simulink model "ThdRwLtStBkReclnIsPosChk"  (R2024b)
settings: Solver=FixedStepDiscrete  StartTime=0.0  StopTime=10.0  FixedStep=0.01  RelTol=1e-3
undefined symbols (not defined in the file or in its folder): KeSMSuThrdRwStBackPosDelta_Val, KeSMSuThrdRwStBackPosTolr_Val, KeSMSuVehicleModelConfig_Val
libraries: StIsPosChkLib x14, simulink x5
(part 1 of 2)
settings Model: Creator=sn2xws  LastModifiedBy=sn55gm
settings Model: ModifiedHistory=|
  | 2024.3.14
  | V2.3.0
  | Bug 813950 童锁Lock，Mode1_Easy Entry Mode 不应调用失败
  | 2024.6.25
  | V3.0.0 557模式流程V1.6
  | 
  | 2024.7.5
  | V3.0.0 557模式流程V1.9
  | 2024.9.5 V3.0.1 新增Md56
  | 2024.10.14 V3.0.2 新增Md57 Md58
  | 2024.10.28 V3.0.3 6s不选Md12目标位置
  | 2024.11.11 V3.0.4 vip模式到位置不看三排
  | 2024.12.24 V3.8.0 CR960542 7s智享退出模式左右同时调用时，三排座椅前后记忆位置使用逻辑
  | 2025.2.19 V3.8.1 Bug 991386 Md1 三排占座时未移动且报了成功
  | 25.6.30 V3.13.0 新增Md61 md62
settings SolverCC: AlgebraicLoopSolver=TrustRegion
settings DataIOCC: SaveFormat=StructureWithTime  ReturnWorkspaceOutputs=off
settings OptimizationCC: DefaultParameterBehavior=Inlined  EnhancedBackFolding=on  PassReuseOutputArgsAs=Individual arguments  ZeroExternalMemoryAtStartup=off  ZeroInternalMemoryAtStartup=off  OptimizeBlockOrder=speed  DifferentSizesBufferReuse=on  OptimizationCustomize=off  EfficientTunableParamExpr=on
settings DebuggingCC: ParameterTunabilityLossMsg=error  UnconnectedInputMsg=warning  UnconnectedOutputMsg=warning  UnconnectedLineMsg=warning  ArithmeticOperatorsInVariantConditions=warning
settings ModelReferenceCC: EnableRefExpFcnMdlSchedulingChecks=on  ModelReferenceNumInstancesAllowed=Single
settings SFSimCC: MATLABDynamicMemAlloc=off  CustomCodeUndefinedFunction=UseInterfaceOnly
settings RTWCC: Description=AUTOSAR  SystemTargetFile=autosar.tlc  GenCodeOnly=on  TemplateMakefile=ert_default_tmf  GenerateReport=on  IncludeHyperlinkInReport=on  LaunchReport=on  DataTypeReplacement=CDataTypesFixedWidth  GenerateTraceInfo=on  GenerateTraceReport=on  GenerateTraceReportSl=on  GenerateTraceReportSf=on  GenerateTraceReportEml=on  GPUComputeCapability=3.5
settings CodeAppCC: ForceParamTrailComments=on  IgnoreCustomStorageClasses=off  OperatorAnnotations=on  SimulinkDataObjDesc=on  SFDataObjDesc=on  InsertBlockDesc=on
settings STFCustomTargetCC: TargetLangStandard=C99 (ISO)  MultiwordLength=256  ParMdlRefBuildCompliant=on  CompOptLevelCompliant=on  IncludeMdlTerminateFcn=off  CombineOutputUpdateFcns=on  SuppressErrorStatus=on  ERTCustomFileBanners=on  SupportNonFinite=off  SupportComplex=off  SupportContinuousTime=off  SupportNonInlinedSFcns=off  RemoveResetFunc=on  MATLABClassNameForMDSCustomization=Simulink.SoftwareTarget.ERTCustomization  AutosarCompliant=on  UseToolchainInfoCompliant=on  LookupTableObjectStructAxisOrder=2,1,3,4,...  LUTObjectStructOrderEvenSpacing=Size,Table,Breakpoints  SystemTargetFile=autosar.tlc
settings ERTTargetCC: TargetLangStandard=C99 (ISO)  ConcurrentExecutionCompliant=off  IncludeMdlTerminateFcn=off  SuppressErrorStatus=on  SupportNonFinite=off  SupportComplex=off  ModelStepFunctionPrototypeControlCompliant=off  CPPClassGenCompliant=off  AutosarCompliant=on  LookupTableObjectStructAxisOrder=2,1,3,4,...  LUTObjectStructOrderEvenSpacing=Size,Table,Breakpoints  ERTCustomFileTemplate=example_file_process.tlc  ERTFilePackagingFormat=Compact  BooleanTrueId=TRUE  BooleanFalseId=FALSE  DynamicArrayContainerType=coder::array

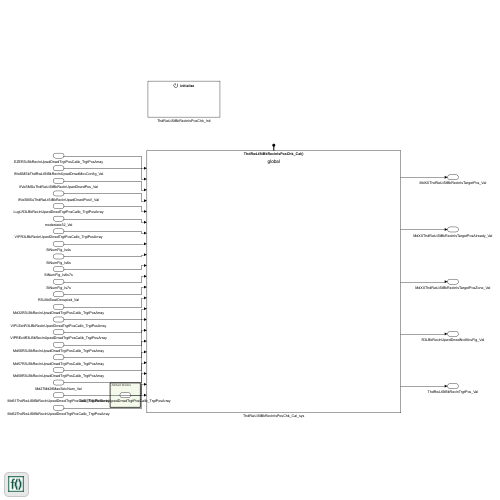
[thumbnail: Simulink's stored preview of the top-level diagram]
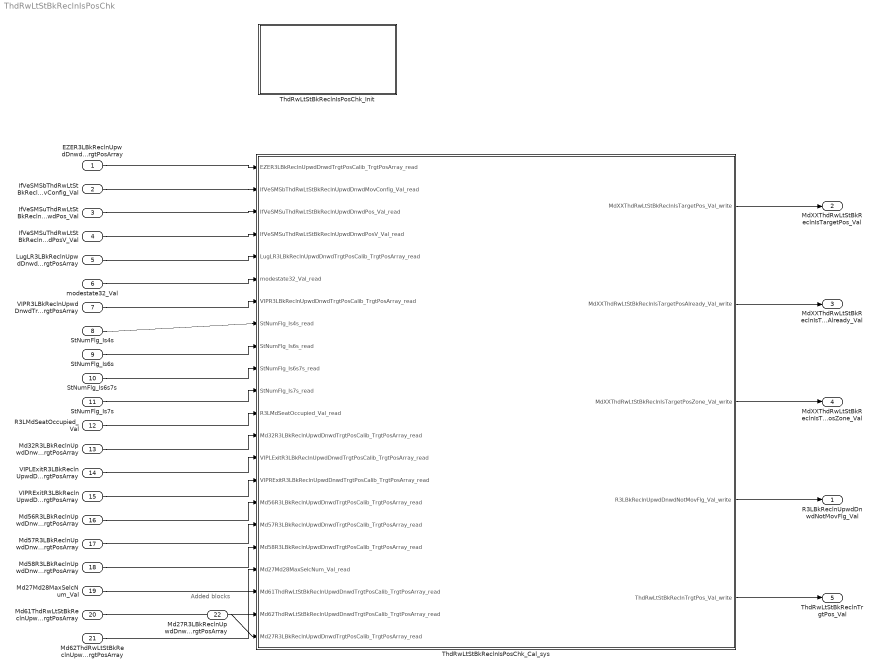
== system ThdRwLtStBkReclnIsPosChk ==
  note: Added blocks
  EZER3LBkReclnUpwdDnwdTrgtPosCalib_TrgtPosArray : Inport  Description=|  OutDataTypeStr=uint16  PortDimensions=3
      | 0:Pos
      | 1:Max
      | 2:Min
  IfVeSMSbThdRwLtStBkReclnUpwdDnwdMovConfig_Val : Inport  Port=2  OutDataTypeStr=boolean  PortDimensions=1
  IfVeSMSuThdRwLtStBkReclnUpwdDnwdPos_Val : Inport  Port=3  OutDataTypeStr=uint16  PortDimensions=1
  IfVeSMSuThdRwLtStBkReclnUpwdDnwdPosV_Val : Inport  Port=4  OutDataTypeStr=boolean  PortDimensions=1
  LugLR3LBkReclnUpwdDnwdTrgtPosCalib_TrgtPosArray : Inport  Description=|  Port=5  OutDataTypeStr=uint16  PortDimensions=3
      | 0:Pos
      | 1:Max
      | 2:Min
  modestate32_Val : Inport  Port=6  OutDataTypeStr=uint32  PortDimensions=1
  VIPR3LBkReclnUpwdDnwdTrgtPosCalib_TrgtPosArray : Inport  Description=|  Port=7  OutDataTypeStr=uint16  PortDimensions=3
      | 0:Pos
      | 1:Max
      | 2:Min
  StNumFlg_Is4s : Inport  Port=8  OutDataTypeStr=boolean  PortDimensions=1
  StNumFlg_Is6s : Inport  Port=9  OutDataTypeStr=boolean  PortDimensions=1
  StNumFlg_Is6s7s : Inport  Port=10  OutDataTypeStr=boolean  PortDimensions=1
  StNumFlg_Is7s : Inport  Port=11  OutDataTypeStr=boolean  PortDimensions=1
  R3LMdSeatOccupied_Val : Inport  Port=12  OutDataTypeStr=boolean  PortDimensions=1
  Md32R3LBkReclnUpwdDnwdTrgtPosCalib_TrgtPosArray : Inport  Description=|  Port=13  OutDataTypeStr=uint16  PortDimensions=3
      | 0:Pos
      | 1:Max
      | 2:Min
  VIPLExitR3LBkReclnUpwdDnwdTrgtPosCalib_TrgtPosArray : Inport  Description=|  Port=14  OutDataTypeStr=uint16  PortDimensions=3
      | 0:Pos
      | 1:Max
      | 2:Min
  VIPRExitR3LBkReclnUpwdDnwdTrgtPosCalib_TrgtPosArray : Inport  Description=|  Port=15  OutDataTypeStr=uint16  PortDimensions=3
      | 0:Pos
      | 1:Max
      | 2:Min
  Md56R3LBkReclnUpwdDnwdTrgtPosCalib_TrgtPosArray : Inport  Description=|  Port=16  OutDataTypeStr=uint16  PortDimensions=3
      | 0:Pos
      | 1:Max
      | 2:Min
  Md57R3LBkReclnUpwdDnwdTrgtPosCalib_TrgtPosArray : Inport  Description=|  Port=17  OutDataTypeStr=uint16  PortDimensions=3
      | 0:Pos
      | 1:Max
      | 2:Min
  Md58R3LBkReclnUpwdDnwdTrgtPosCalib_TrgtPosArray : Inport  Description=|  Port=18  OutDataTypeStr=uint16  PortDimensions=3
      | 0:Pos
      | 1:Max
      | 2:Min
  Md27Md28MaxSelcNum_Val : Inport  Port=19  OutDataTypeStr=uint8  PortDimensions=1
  Md61ThdRwLtStBkReclnUpwdDnwdTrgtPosCalib_TrgtPosArray : Inport  Description=|  Port=20  OutDataTypeStr=uint16  PortDimensions=3
      | 0:Pos
      | 1:Max
      | 2:Min
  Md62ThdRwLtStBkReclnUpwdDnwdTrgtPosCalib_TrgtPosArray : Inport  Description=|  Port=21  OutDataTypeStr=uint16  PortDimensions=3
      | 0:Pos
      | 1:Max
      | 2:Min
  Md27R3LBkReclnUpwdDnwdTrgtPosCalib_TrgtPosArray : Inport  Description=|  Port=22  OutDataTypeStr=uint16  PortDimensions=3
      | 0:Pos
      | 1:Max
      | 2:Min
  ThdRwLtStBkReclnIsPosChk_Cal_sys : Subsystem
  ThdRwLtStBkReclnIsPosChk_Init : Subsystem
  R3LBkReclnUpwdDnwdNotMovFlg_Val : Outport  OutDataTypeStr=boolean  PortDimensions=1  VectorParamsAs1DForOutWhenUnconnected=off
  MdXXThdRwLtStBkReclnIsTargetPos_Val : Outport  Port=2  OutDataTypeStr=uint32  PortDimensions=1  VectorParamsAs1DForOutWhenUnconnected=off
  MdXXThdRwLtStBkReclnIsTargetPosAlready_Val : Outport  Port=3  OutDataTypeStr=uint32  PortDimensions=1  VectorParamsAs1DForOutWhenUnconnected=off
  MdXXThdRwLtStBkReclnIsTargetPosZone_Val : Outport  Port=4  OutDataTypeStr=uint32  PortDimensions=1  VectorParamsAs1DForOutWhenUnconnected=off
  ThdRwLtStBkReclnTrgtPos_Val : Outport  Port=5  OutDataTypeStr=uint16  PortDimensions=1  VectorParamsAs1DForOutWhenUnconnected=off
  wires:
  EZER3LBkReclnUpwdDnwdTrgtPosCalib_TrgtPosArray/1 -> ThdRwLtStBkReclnIsPosChk_Cal_sys/1(EZER3LBkReclnUpwdDnwdTrgtPosCalib_TrgtPosArray_read)
  IfVeSMSbThdRwLtStBkReclnUpwdDnwdMovConfig_Val/1 -> ThdRwLtStBkReclnIsPosChk_Cal_sys/2(IfVeSMSbThdRwLtStBkReclnUpwdDnwdMovConfig_Val_read)
  IfVeSMSuThdRwLtStBkReclnUpwdDnwdPos_Val/1 -> ThdRwLtStBkReclnIsPosChk_Cal_sys/3(IfVeSMSuThdRwLtStBkReclnUpwdDnwdPos_Val_read)
  IfVeSMSuThdRwLtStBkReclnUpwdDnwdPosV_Val/1 -> ThdRwLtStBkReclnIsPosChk_Cal_sys/4(IfVeSMSuThdRwLtStBkReclnUpwdDnwdPosV_Val_read)
  LugLR3LBkReclnUpwdDnwdTrgtPosCalib_TrgtPosArray/1 -> ThdRwLtStBkReclnIsPosChk_Cal_sys/5(LugLR3LBkReclnUpwdDnwdTrgtPosCalib_TrgtPosArray_read)
  modestate32_Val/1 -> ThdRwLtStBkReclnIsPosChk_Cal_sys/6(modestate32_Val_read)
  VIPR3LBkReclnUpwdDnwdTrgtPosCalib_TrgtPosArray/1 -> ThdRwLtStBkReclnIsPosChk_Cal_sys/7(VIPR3LBkReclnUpwdDnwdTrgtPosCalib_TrgtPosArray_read)
  ThdRwLtStBkReclnIsPosChk_Cal_sys/1(MdXXThdRwLtStBkReclnIsTargetPos_Val_write) -> MdXXThdRwLtStBkReclnIsTargetPos_Val/1
  ThdRwLtStBkReclnIsPosChk_Cal_sys/2(MdXXThdRwLtStBkReclnIsTargetPosAlready_Val_write) -> MdXXThdRwLtStBkReclnIsTargetPosAlready_Val/1
  ThdRwLtStBkReclnIsPosChk_Cal_sys/3(MdXXThdRwLtStBkReclnIsTargetPosZone_Val_write) -> MdXXThdRwLtStBkReclnIsTargetPosZone_Val/1
  ThdRwLtStBkReclnIsPosChk_Cal_sys/4(R3LBkReclnUpwdDnwdNotMovFlg_Val_write) -> R3LBkReclnUpwdDnwdNotMovFlg_Val/1
  ThdRwLtStBkReclnIsPosChk_Cal_sys/5(ThdRwLtStBkReclnTrgtPos_Val_write) -> ThdRwLtStBkReclnTrgtPos_Val/1
  StNumFlg_Is4s/1 -> ThdRwLtStBkReclnIsPosChk_Cal_sys/8(StNumFlg_Is4s_read)
  StNumFlg_Is6s/1 -> ThdRwLtStBkReclnIsPosChk_Cal_sys/9(StNumFlg_Is6s_read)
  StNumFlg_Is6s7s/1 -> ThdRwLtStBkReclnIsPosChk_Cal_sys/10(StNumFlg_Is6s7s_read)
  StNumFlg_Is7s/1 -> ThdRwLtStBkReclnIsPosChk_Cal_sys/11(StNumFlg_Is7s_read)
  R3LMdSeatOccupied_Val/1 -> ThdRwLtStBkReclnIsPosChk_Cal_sys/12(R3LMdSeatOccupied_Val_read)
  Md32R3LBkReclnUpwdDnwdTrgtPosCalib_TrgtPosArray/1 -> ThdRwLtStBkReclnIsPosChk_Cal_sys/13(Md32R3LBkReclnUpwdDnwdTrgtPosCalib_TrgtPosArray_read)
  VIPLExitR3LBkReclnUpwdDnwdTrgtPosCalib_TrgtPosArray/1 -> ThdRwLtStBkReclnIsPosChk_Cal_sys/14(VIPLExitR3LBkReclnUpwdDnwdTrgtPosCalib_TrgtPosArray_read)
  VIPRExitR3LBkReclnUpwdDnwdTrgtPosCalib_TrgtPosArray/1 -> ThdRwLtStBkReclnIsPosChk_Cal_sys/15(VIPRExitR3LBkReclnUpwdDnwdTrgtPosCalib_TrgtPosArray_read)
  Md56R3LBkReclnUpwdDnwdTrgtPosCalib_TrgtPosArray/1 -> ThdRwLtStBkReclnIsPosChk_Cal_sys/16(Md56R3LBkReclnUpwdDnwdTrgtPosCalib_TrgtPosArray_read)
  Md57R3LBkReclnUpwdDnwdTrgtPosCalib_TrgtPosArray/1 -> ThdRwLtStBkReclnIsPosChk_Cal_sys/17(Md57R3LBkReclnUpwdDnwdTrgtPosCalib_TrgtPosArray_read)
  Md58R3LBkReclnUpwdDnwdTrgtPosCalib_TrgtPosArray/1 -> ThdRwLtStBkReclnIsPosChk_Cal_sys/18(Md58R3LBkReclnUpwdDnwdTrgtPosCalib_TrgtPosArray_read)
  Md27Md28MaxSelcNum_Val/1 -> ThdRwLtStBkReclnIsPosChk_Cal_sys/19(Md27Md28MaxSelcNum_Val_read)
  Md61ThdRwLtStBkReclnUpwdDnwdTrgtPosCalib_TrgtPosArray/1 -> ThdRwLtStBkReclnIsPosChk_Cal_sys/20(Md61ThdRwLtStBkReclnUpwdDnwdTrgtPosCalib_TrgtPosArray_read)
  Md62ThdRwLtStBkReclnUpwdDnwdTrgtPosCalib_TrgtPosArray/1 -> ThdRwLtStBkReclnIsPosChk_Cal_sys/21(Md62ThdRwLtStBkReclnUpwdDnwdTrgtPosCalib_TrgtPosArray_read)
  Md27R3LBkReclnUpwdDnwdTrgtPosCalib_TrgtPosArray/1 -> ThdRwLtStBkReclnIsPosChk_Cal_sys/22(Md27R3LBkReclnUpwdDnwdTrgtPosCalib_TrgtPosArray_read)

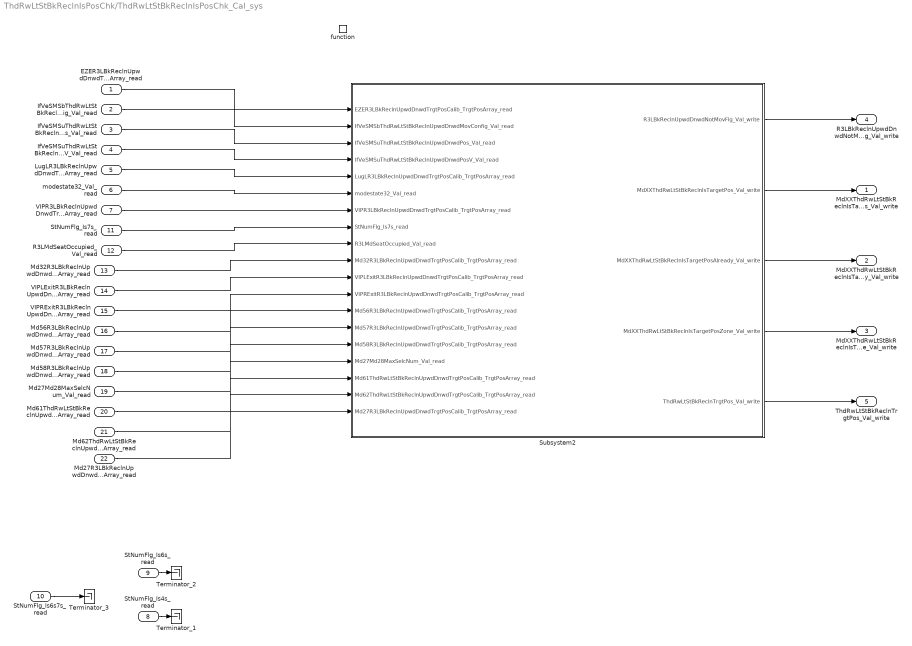
== system ThdRwLtStBkReclnIsPosChk/ThdRwLtStBkReclnIsPosChk_Cal_sys ==
  EZER3LBkReclnUpwdDnwdTrgtPosCalib_TrgtPosArray_read : Inport
  IfVeSMSbThdRwLtStBkReclnUpwdDnwdMovConfig_Val_read : Inport  Port=2
  IfVeSMSuThdRwLtStBkReclnUpwdDnwdPos_Val_read : Inport  Port=3
  IfVeSMSuThdRwLtStBkReclnUpwdDnwdPosV_Val_read : Inport  Port=4
  LugLR3LBkReclnUpwdDnwdTrgtPosCalib_TrgtPosArray_read : Inport  Port=5
  modestate32_Val_read : Inport  Port=6
  VIPR3LBkReclnUpwdDnwdTrgtPosCalib_TrgtPosArray_read : Inport  Port=7
  StNumFlg_Is4s_read : Inport  Port=8
  StNumFlg_Is6s_read : Inport  Port=9
  StNumFlg_Is6s7s_read : Inport  Port=10
  StNumFlg_Is7s_read : Inport  Port=11
  R3LMdSeatOccupied_Val_read : Inport  Port=12
  Md32R3LBkReclnUpwdDnwdTrgtPosCalib_TrgtPosArray_read : Inport  Port=13
  VIPLExitR3LBkReclnUpwdDnwdTrgtPosCalib_TrgtPosArray_read : Inport  Port=14
  VIPRExitR3LBkReclnUpwdDnwdTrgtPosCalib_TrgtPosArray_read : Inport  Port=15
  Md56R3LBkReclnUpwdDnwdTrgtPosCalib_TrgtPosArray_read : Inport  Port=16
  Md57R3LBkReclnUpwdDnwdTrgtPosCalib_TrgtPosArray_read : Inport  Port=17
  Md58R3LBkReclnUpwdDnwdTrgtPosCalib_TrgtPosArray_read : Inport  Port=18
  Md27Md28MaxSelcNum_Val_read : Inport  Port=19
  Md61ThdRwLtStBkReclnUpwdDnwdTrgtPosCalib_TrgtPosArray_read : Inport  Port=20
  Md62ThdRwLtStBkReclnUpwdDnwdTrgtPosCalib_TrgtPosArray_read : Inport  Port=21
  Md27R3LBkReclnUpwdDnwdTrgtPosCalib_TrgtPosArray_read : Inport  Port=22
  function : TriggerPort  TriggerType=function-call  IsSimulinkFunction=on  FunctionName=ThdRwLtStBkReclnIsPosChk_Cal  VariantControl=(inherit)
  Subsystem2 : Subsystem
  Terminator_1 : Terminator
  Terminator_2 : Terminator
  Terminator_3 : Terminator
  MdXXThdRwLtStBkReclnIsTargetPos_Val_write : Outport  VectorParamsAs1DForOutWhenUnconnected=off
      settings: EnsureOutportIsVirtual=on
  MdXXThdRwLtStBkReclnIsTargetPosAlready_Val_write : Outport  Port=2  VectorParamsAs1DForOutWhenUnconnected=off
      settings: EnsureOutportIsVirtual=on
  MdXXThdRwLtStBkReclnIsTargetPosZone_Val_write : Outport  Port=3  VectorParamsAs1DForOutWhenUnconnected=off
      settings: EnsureOutportIsVirtual=on
  R3LBkReclnUpwdDnwdNotMovFlg_Val_write : Outport  Port=4  VectorParamsAs1DForOutWhenUnconnected=off
      settings: EnsureOutportIsVirtual=on
  ThdRwLtStBkReclnTrgtPos_Val_write : Outport  Port=5  VectorParamsAs1DForOutWhenUnconnected=off
      settings: EnsureOutportIsVirtual=on
  wires:
  Subsystem2/1(R3LBkReclnUpwdDnwdNotMovFlg_Val_write) -> R3LBkReclnUpwdDnwdNotMovFlg_Val_write/1
  Subsystem2/2(MdXXThdRwLtStBkReclnIsTargetPos_Val_write) -> MdXXThdRwLtStBkReclnIsTargetPos_Val_write/1
  Subsystem2/3(MdXXThdRwLtStBkReclnIsTargetPosAlready_Val_write) -> MdXXThdRwLtStBkReclnIsTargetPosAlready_Val_write/1
  Subsystem2/4(MdXXThdRwLtStBkReclnIsTargetPosZone_Val_write) -> MdXXThdRwLtStBkReclnIsTargetPosZone_Val_write/1
  Subsystem2/5(ThdRwLtStBkReclnTrgtPos_Val_write) -> ThdRwLtStBkReclnTrgtPos_Val_write/1
  IfVeSMSuThdRwLtStBkReclnUpwdDnwdPos_Val_read/1 -> Subsystem2/3(IfVeSMSuThdRwLtStBkReclnUpwdDnwdPos_Val_read)
  IfVeSMSbThdRwLtStBkReclnUpwdDnwdMovConfig_Val_read/1 -> Subsystem2/2(IfVeSMSbThdRwLtStBkReclnUpwdDnwdMovConfig_Val_read)
  EZER3LBkReclnUpwdDnwdTrgtPosCalib_TrgtPosArray_read/1 -> Subsystem2/1(EZER3LBkReclnUpwdDnwdTrgtPosCalib_TrgtPosArray_read)
  IfVeSMSuThdRwLtStBkReclnUpwdDnwdPosV_Val_read/1 -> Subsystem2/4(IfVeSMSuThdRwLtStBkReclnUpwdDnwdPosV_Val_read)
  LugLR3LBkReclnUpwdDnwdTrgtPosCalib_TrgtPosArray_read/1 -> Subsystem2/5(LugLR3LBkReclnUpwdDnwdTrgtPosCalib_TrgtPosArray_read)
  modestate32_Val_read/1 -> Subsystem2/6(modestate32_Val_read)
  VIPR3LBkReclnUpwdDnwdTrgtPosCalib_TrgtPosArray_read/1 -> Subsystem2/7(VIPR3LBkReclnUpwdDnwdTrgtPosCalib_TrgtPosArray_read)
  StNumFlg_Is4s_read/1 -> Terminator_1/1
  StNumFlg_Is6s7s_read/1 -> Terminator_3/1
  StNumFlg_Is7s_read/1 -> Subsystem2/8(StNumFlg_Is7s_read)
  StNumFlg_Is6s_read/1 -> Terminator_2/1
  R3LMdSeatOccupied_Val_read/1 -> Subsystem2/9(R3LMdSeatOccupied_Val_read)
  Md32R3LBkReclnUpwdDnwdTrgtPosCalib_TrgtPosArray_read/1 -> Subsystem2/10(Md32R3LBkReclnUpwdDnwdTrgtPosCalib_TrgtPosArray_read)
  VIPLExitR3LBkReclnUpwdDnwdTrgtPosCalib_TrgtPosArray_read/1 -> Subsystem2/11(VIPLExitR3LBkReclnUpwdDnwdTrgtPosCalib_TrgtPosArray_read)
  VIPRExitR3LBkReclnUpwdDnwdTrgtPosCalib_TrgtPosArray_read/1 -> Subsystem2/12(VIPRExitR3LBkReclnUpwdDnwdTrgtPosCalib_TrgtPosArray_read)
  Md56R3LBkReclnUpwdDnwdTrgtPosCalib_TrgtPosArray_read/1 -> Subsystem2/13(Md56R3LBkReclnUpwdDnwdTrgtPosCalib_TrgtPosArray_read)
  Md57R3LBkReclnUpwdDnwdTrgtPosCalib_TrgtPosArray_read/1 -> Subsystem2/14(Md57R3LBkReclnUpwdDnwdTrgtPosCalib_TrgtPosArray_read)
  Md58R3LBkReclnUpwdDnwdTrgtPosCalib_TrgtPosArray_read/1 -> Subsystem2/15(Md58R3LBkReclnUpwdDnwdTrgtPosCalib_TrgtPosArray_read)
  Md27Md28MaxSelcNum_Val_read/1 -> Subsystem2/16(Md27Md28MaxSelcNum_Val_read)
  Md61ThdRwLtStBkReclnUpwdDnwdTrgtPosCalib_TrgtPosArray_read/1 -> Subsystem2/17(Md61ThdRwLtStBkReclnUpwdDnwdTrgtPosCalib_TrgtPosArray_read)
  Md62ThdRwLtStBkReclnUpwdDnwdTrgtPosCalib_TrgtPosArray_read/1 -> Subsystem2/18(Md62ThdRwLtStBkReclnUpwdDnwdTrgtPosCalib_TrgtPosArray_read)
  Md27R3LBkReclnUpwdDnwdTrgtPosCalib_TrgtPosArray_read/1 -> Subsystem2/19(Md27R3LBkReclnUpwdDnwdTrgtPosCalib_TrgtPosArray_read)

== system ThdRwLtStBkReclnIsPosChk/ThdRwLtStBkReclnIsPosChk_Init ==
  note: Added blocks
  note: Added blocks
  note: Added blocks
  Event Listener : EventListener  EventName=reset
  PA_KeSMSuThrdRwStBackPosDelta_Val : Constant  Value=KeSMSuThrdRwStBackPosDelta_Val
  PA_KeSMSuThrdRwStBackPosTolr_Val : Constant  Value=KeSMSuThrdRwStBackPosTolr_Val
  PA_KeSMSuVehicleModelConfig_Val : Constant  Value=KeSMSuVehicleModelConfig_Val
  Terminator_1 : Terminator
  Terminator_2 : Terminator
  Terminator_3 : Terminator
  wires:
  PA_KeSMSuThrdRwStBackPosDelta_Val/1 -> Terminator_1/1
  PA_KeSMSuThrdRwStBackPosTolr_Val/1 -> Terminator_2/1
  PA_KeSMSuVehicleModelConfig_Val/1 -> Terminator_3/1

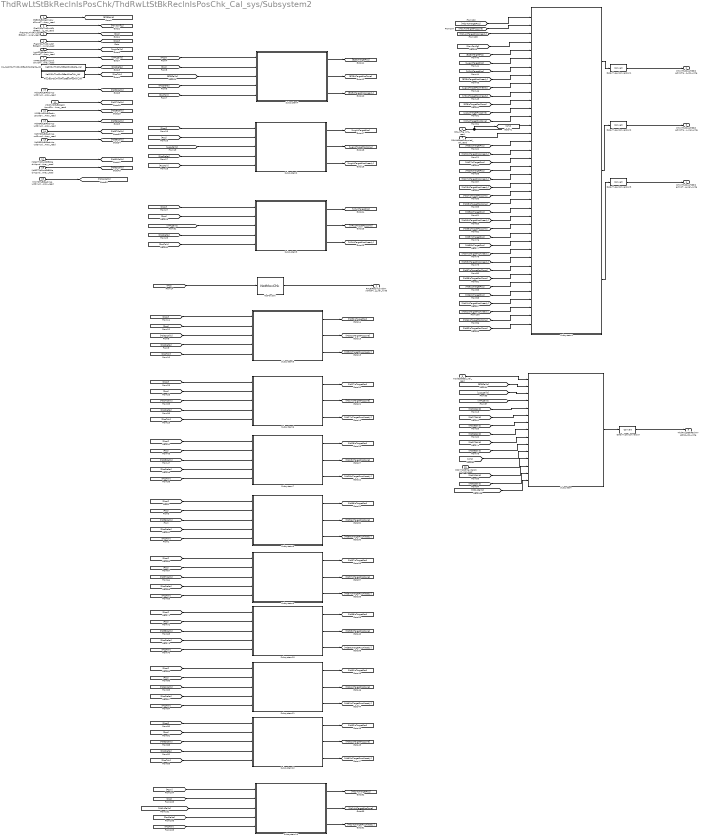
== system ThdRwLtStBkReclnIsPosChk/ThdRwLtStBkReclnIsPosChk_Cal_sys/Subsystem2 ==
  EZER3LBkReclnUpwdDnwdTrgtPosCalib_TrgtPosArray_read : Inport
  IfVeSMSbThdRwLtStBkReclnUpwdDnwdMovConfig_Val_read : Inport  Port=2
  IfVeSMSuThdRwLtStBkReclnUpwdDnwdPos_Val_read : Inport  Port=3
  IfVeSMSuThdRwLtStBkReclnUpwdDnwdPosV_Val_read : Inport  Port=4
  LugLR3LBkReclnUpwdDnwdTrgtPosCalib_TrgtPosArray_read : Inport  Port=5
  modestate32_Val_read : Inport  Port=6
  VIPR3LBkReclnUpwdDnwdTrgtPosCalib_TrgtPosArray_read : Inport  Port=7
  StNumFlg_Is7s_read : Inport  Port=8
  R3LMdSeatOccupied_Val_read : Inport  Port=9
  Md32R3LBkReclnUpwdDnwdTrgtPosCalib_TrgtPosArray_read : Inport  Port=10
  VIPLExitR3LBkReclnUpwdDnwdTrgtPosCalib_TrgtPosArray_read : Inport  Port=11
  VIPRExitR3LBkReclnUpwdDnwdTrgtPosCalib_TrgtPosArray_read : Inport  Port=12
  Md56R3LBkReclnUpwdDnwdTrgtPosCalib_TrgtPosArray_read : Inport  Port=13
  Md57R3LBkReclnUpwdDnwdTrgtPosCalib_TrgtPosArray_read : Inport  Port=14
  Md58R3LBkReclnUpwdDnwdTrgtPosCalib_TrgtPosArray_read : Inport  Port=15
  Md27Md28MaxSelcNum_Val_read : Inport  Port=16
  Md61ThdRwLtStBkReclnUpwdDnwdTrgtPosCalib_TrgtPosArray_read : Inport  Port=17
  Md62ThdRwLtStBkReclnUpwdDnwdTrgtPosCalib_TrgtPosArray_read : Inport  Port=18
  Md27R3LBkReclnUpwdDnwdTrgtPosCalib_TrgtPosArray_read : Inport  Port=19
  Data Type Conversion{,1..3} (4 alike) : DataTypeConversion  SaturateOnIntegerOverflow=off  RndMeth=Floor
  NotMovChk : StIsPosChkLib/NotMovChk  SystemSampleTime=-1  VariantActivationTime=update diagram  AllowFlexibleInterface=on  Latency=0  AutoFrameSizeCalculation=off
  PA_KeSMSuThrdRwStBackPosDelta_Val : Constant  Value=KeSMSuThrdRwStBackPosDelta_Val
  PA_KeSMSuThrdRwStBackPosTolr_Val : Constant  Value=KeSMSuThrdRwStBackPosTolr_Val
  Subsystem : Subsystem
  Subsystem1 : Subsystem
  Subsystem10 : Subsystem
  Subsystem11 : Subsystem
  Subsystem12 : Subsystem
  Subsystem13 : Subsystem
  Subsystem2 : Subsystem
  Subsystem3 : Subsystem
  Subsystem4 : Subsystem
  Subsystem5 : Subsystem
  Subsystem6 : Subsystem
  Subsystem7 : Subsystem
  Subsystem8 : Subsystem
  Subsystem9 : Subsystem
  R3LBkReclnUpwdDnwdNotMovFlg_Val_write : Outport  VectorParamsAs1DForOutWhenUnconnected=off
      settings: EnsureOutportIsVirtual=on
  MdXXThdRwLtStBkReclnIsTargetPos_Val_write : Outport  Port=2  VectorParamsAs1DForOutWhenUnconnected=off
      settings: EnsureOutportIsVirtual=on
  MdXXThdRwLtStBkReclnIsTargetPosAlready_Val_write : Outport  Port=3  VectorParamsAs1DForOutWhenUnconnected=off
      settings: EnsureOutportIsVirtual=on
  MdXXThdRwLtStBkReclnIsTargetPosZone_Val_write : Outport  Port=4  VectorParamsAs1DForOutWhenUnconnected=off
      settings: EnsureOutportIsVirtual=on
  ThdRwLtStBkReclnTrgtPos_Val_write : Outport  Port=5  VectorParamsAs1DForOutWhenUnconnected=off
      settings: EnsureOutportIsVirtual=on
  wires:
  Subsystem4/2(IsPosZone) -> [EZEIsTargetPosZone]
  Subsystem4/3(IsPosAlready) -> [EZEIsTargetPosAlready]
  [LugLCalib] -> Subsystem2/3(CalibArray)
  [PosDelta] -> Subsystem3/4(Delta)
  Subsystem2/1(IsPos) -> [LugLIsTargetPos]
  [PosV] -> Subsystem4/1(PosV)
  [VIPLIsTargetPosZone] -> Subsystem1/13(VIPLIsTargetPosZone)
  [Pos] -> Subsystem4/2(Pos)
  [PosV] -> Subsystem3/1(PosV)
  [PosDelta] -> Subsystem2/4(Delta)
  Subsystem/1(TrgtPos) -> Data Type Conversion/1
  IfVeSMSuThdRwLtStBkReclnUpwdDnwdPos_Val_read/1 -> [Pos]
  [LugLIsTargetPos] -> Subsystem1/6(LugLIsTargetPos)
  modestate32_Val_read/1 -> Subsystem/1(modestate32_Val_read)
  Subsystem3/1(IsPos) -> [VIPLIsTargetPos]
  Subsystem4/1(IsPos) -> [EZEIsTargetPos]
  [VIPLIsTargetPosAlready] -> Subsystem1/10(VIPLIsTargetPosAlready)
  [Pos] -> Subsystem2/2(Pos)
  Subsystem3/2(IsPosZone) -> [VIPLIsTargetPosZone]
  [EZEIsTargetPosAlready] -> Subsystem1/8(EZEIsTargetPosAlready)
  [VIPLCalib] -> Subsystem3/3(CalibArray)
  EZER3LBkReclnUpwdDnwdTrgtPosCalib_TrgtPosArray_read/1 -> [EZECalib]
  Subsystem1/1(IsTargetPos) -> Data Type Conversion1/1
  [EZECalib] -> Subsystem/2(EZECalib)
  [PosTolr] -> Subsystem4/5(Tolr)
  [EZEIsTargetPosZone] -> Subsystem1/11(EZEIsTargetPosZone)
  [PosDelta] -> Subsystem4/4(Delta)
  [MovConfig] -> Subsystem1/4(MovConfig)
  PA_KeSMSuThrdRwStBackPosDelta_Val/1 -> [PosDelta]
  [PosTolr] -> Subsystem2/5(Tolr)
  LugLR3LBkReclnUpwdDnwdTrgtPosCalib_TrgtPosArray_read/1 -> [LugLCalib]
  Subsystem1/2(IsTargetPosAlready) -> Data Type Conversion2/1
  NotMovChk/1 -> R3LBkReclnUpwdDnwdNotMovFlg_Val_write/1
  Subsystem3/3(IsPosAlready) -> [VIPLIsTargetPosAlready]
  [EZEIsTargetPos] -> Subsystem1/5(EZEIsTargetPos)
  Data Type Conversion/1 -> ThdRwLtStBkReclnTrgtPos_Val_write/1
  [LugLIsTargetPosAlready] -> Subsystem1/9(LugLIsTargetPosAlready)
  [LugLIsTargetPosZone] -> Subsystem1/12(LugLIsTargetPosZone)
  [VIPLCalib] -> Subsystem/4(VIPLCalib)
  Subsystem2/3(IsPosAlready) -> [LugLIsTargetPosAlready]
  Data Type Conversion3/1 -> MdXXThdRwLtStBkReclnIsTargetPosZone_Val_write/1
  VIPR3LBkReclnUpwdDnwdTrgtPosCalib_TrgtPosArray_read/1 -> [VIPLCalib]
  [EZECalib] -> Subsystem4/3(CalibArray)
  [VIPLIsTargetPos] -> Subsystem1/7(VIPLIsTargetPos)
  [Pos] -> NotMovChk/1
  Data Type Conversion1/1 -> MdXXThdRwLtStBkReclnIsTargetPos_Val_write/1
  IfVeSMSuThdRwLtStBkReclnUpwdDnwdPosV_Val_read/1 -> [PosV]
  [PosV] -> Subsystem2/1(PosV)
  Subsystem1/3(IsTargetPosZone) -> Data Type Conversion3/1
  PA_KeSMSuThrdRwStBackPosTolr_Val/1 -> [PosTolr]
  Data Type Conversion2/1 -> MdXXThdRwLtStBkReclnIsTargetPosAlready_Val_write/1
  IfVeSMSbThdRwLtStBkReclnUpwdDnwdMovConfig_Val_read/1 -> [MovConfig]
  [Pos] -> Subsystem3/2(Pos)
  Subsystem2/2(IsPosZone) -> [LugLIsTargetPosZone]
  [PosTolr] -> Subsystem3/5(Tolr)
  [LugLCalib] -> Subsystem/3(EZQCalib)
  StNumFlg_Is7s_read/1 -> [is7s], Subsystem1/14(StNumFlg_Is7s_read)
  R3LMdSeatOccupied_Val_read/1 -> Subsystem1/15(R3LMdSeatOccupied_Val_read)
  Md32R3LBkReclnUpwdDnwdTrgtPosCalib_TrgtPosArray_read/1 -> [Md32Calib]
  [Md32Calib] -> Subsystem5/3(CalibArray)
  [PosTolr] -> Subsystem5/5(Tolr)
  [PosDelta] -> Subsystem5/4(Delta)
  [Pos] -> Subsystem5/2(Pos)
  [PosV] -> Subsystem5/1(PosV)
  Subsystem5/3(IsPosAlready) -> [Md32IsTargetPosAlready]
  Subsystem5/2(IsPosZone) -> [Md32IsTargetPosZone]
  Subsystem5/1(IsPos) -> [Md32IsTargetPos]
  [Md32Calib] -> Subsystem/5(Md32Calib)
  [Md32IsTargetPos] -> Subsystem1/16(Md32IsTargetPos)
  [Md32IsTargetPosAlready] -> Subsystem1/17(Md32IsTargetPosAlready)
  [PosV] -> Subsystem6/1(PosV)
  [Pos] -> Subsystem6/2(Pos)
  [PosDelta] -> Subsystem6/4(Delta)
  [PosTolr] -> Subsystem6/5(Tolr)
  [Md27Calib] -> Subsystem6/3(CalibArray)
  [Md28Calib] -> Subsystem7/3(CalibArray)
  [PosTolr] -> Subsystem7/5(Tolr)
  [PosDelta] -> Subsystem7/4(Delta)
  [Pos] -> Subsystem7/2(Pos)
  [PosV] -> Subsystem7/1(PosV)
  Subsystem6/1(IsPos) -> [Md27IsTargetPos]
  Subsystem6/2(IsPosZone) -> [Md27IsTargetPosZone]
  Subsystem6/3(IsPosAlready) -> [Md27IsTargetPosAlready]
  Subsystem7/3(IsPosAlready) -> [Md28IsTargetPosAlready]
  Subsystem7/2(IsPosZone) -> [Md28IsTargetPosZone]
  Subsystem7/1(IsPos) -> [Md28IsTargetPos]
  [Md27Calib] -> Subsystem/6(Md27Calib)
  [Md28Calib] -> Subsystem/7(Md28Calib)
  [Md27IsTargetPos] -> Subsystem1/18(Md27IsTargetPos)
  [Md27IsTargetPosZone] -> Subsystem1/22(Md27IsTargetPosZone)
  [Md28IsTargetPos] -> Subsystem1/19(Md28IsTargetPos)
  [Md28IsTargetPosZone] -> Subsystem1/23(Md28IsTargetPosZone)
  VIPRExitR3LBkReclnUpwdDnwdTrgtPosCalib_TrgtPosArray_read/1 -> [Md28Calib]
  [Md27IsTargetPosAlready] -> Subsystem1/20(Md27IsTargetPosAlready)
  [Md28IsTargetPosAlready] -> Subsystem1/21(Md28IsTargetPosAlready)
  Md56R3LBkReclnUpwdDnwdTrgtPosCalib_TrgtPosArray_read/1 -> [Md56Calib]
  Subsystem8/1(IsPos) -> [Md56IsTargetPos]
  Subsystem8/2(IsPosZone) -> [Md56IsTargetPosZone]
  Subsystem8/3(IsPosAlready) -> [Md56IsTargetPosAlready]
  [PosV] -> Subsystem8/1(PosV)
  [Pos] -> Subsystem8/2(Pos)
  [PosDelta] -> Subsystem8/4(Delta)
  [PosTolr] -> Subsystem8/5(Tolr)
  [Md56Calib] -> Subsystem8/3(CalibArray)
  [Md56Calib] -> Subsystem/8(Md56Calib)
  [Md56IsTargetPos] -> Subsystem1/24(Md56IsTargetPos)
  [Md56IsTargetPosZone] -> Subsystem1/26(Md56IsTargetPosZone)
  [Md56IsTargetPosAlready] -> Subsystem1/25(Md56IsTargetPosAlready)
  Md58R3LBkReclnUpwdDnwdTrgtPosCalib_TrgtPosArray_read/1 -> [Md58Calib]
  Md57R3LBkReclnUpwdDnwdTrgtPosCalib_TrgtPosArray_read/1 -> [Md57Calib]
  [Md57Calib] -> Subsystem9/3(CalibArray)
  [PosTolr] -> Subsystem9/5(Tolr)
  [PosDelta] -> Subsystem9/4(Delta)
  [Pos] -> Subsystem9/2(Pos)
  [PosV] -> Subsystem9/1(PosV)
  Subsystem9/3(IsPosAlready) -> [Md57IsTargetPosAlready]
  Subsystem9/2(IsPosZone) -> [Md57IsTargetPosZone]
  Subsystem9/1(IsPos) -> [Md57IsTargetPos]
  Subsystem10/1(IsPos) -> [Md58IsTargetPos]
  Subsystem10/2(IsPosZone) -> [Md58IsTargetPosZone]
  Subsystem10/3(IsPosAlready) -> [Md58IsTargetPosAlready]
  [PosV] -> Subsystem10/1(PosV)
  [Pos] -> Subsystem10/2(Pos)
  [PosDelta] -> Subsystem10/4(Delta)
  [PosTolr] -> Subsystem10/5(Tolr)
  [Md58Calib] -> Subsystem10/3(CalibArray)
  [Md58Calib] -> Subsystem/10(Md58Calib)
  [Md57Calib] -> Subsystem/9(Md57Calib)
  [Md57IsTargetPos] -> Subsystem1/27(Md57IsTargetPos)
  [Md58IsTargetPos] -> Subsystem1/28(Md58IsTargetPos)
  [Md57IsTargetPosAlready] -> Subsystem1/29(Md57IsTargetPosAlready)
  [Md58IsTargetPosAlready] -> Subsystem1/30(Md58IsTargetPosAlready)
  [Md57IsTargetPosZone] -> Subsystem1/31(Md57IsTargetPosZone)
  [Md58IsTargetPosZone] -> Subsystem1/32(Md58IsTargetPosZone)
  [is7s] -> Subsystem/11(is7s)
  Md27Md28MaxSelcNum_Val_read/1 -> Subsystem/12(Md27Md28MaxSelcNum_Val_read)
  Md62ThdRwLtStBkReclnUpwdDnwdTrgtPosCalib_TrgtPosArray_read/1 -> [Md62Calib]
  Md61ThdRwLtStBkReclnUpwdDnwdTrgtPosCalib_TrgtPosArray_read/1 -> [Md61Calib]
  [Md61Calib] -> Subsystem11/3(CalibArray)
  [PosTolr] -> Subsystem11/5(Tolr)
  [PosDelta] -> Subsystem11/4(Delta)
  [Pos] -> Subsystem11/2(Pos)
  [PosV] -> Subsystem11/1(PosV)
  Subsystem11/3(IsPosAlready) -> [Md61IsTargetPosAlready]
  Subsystem11/2(IsPosZone) -> [Md61IsTargetPosZone]
  Subsystem11/1(IsPos) -> [Md61IsTargetPos]
  Subsystem12/1(IsPos) -> [Md62IsTargetPos]
  Subsystem12/2(IsPosZone) -> [Md62IsTargetPosZone]
  Subsystem12/3(IsPosAlready) -> [Md62IsTargetPosAlready]
  [PosV] -> Subsystem12/1(PosV)
  [Pos] -> Subsystem12/2(Pos)
  [PosDelta] -> Subsystem12/4(Delta)
  [PosTolr] -> Subsystem12/5(Tolr)
  [Md62Calib] -> Subsystem12/3(CalibArray)
  [Md61Calib] -> Subsystem/13(Md61Calib)
  [Md62Calib] -> Subsystem/14(Md62Calib)
  [Md61IsTargetPos] -> Subsystem1/33(Md61IsTargetPos)
  [Md62IsTargetPos] -> Subsystem1/34(Md62IsTargetPos)
  [Md61IsTargetPosAlready] -> Subsystem1/35(Md61IsTargetPosAlready)
  [Md62IsTargetPosAlready] -> Subsystem1/36(Md62IsTargetPosAlready)
  [Md61IsTargetPosZone] -> Subsystem1/37(Md61IsTargetPosZone)
  [Md62IsTargetPosZone] -> Subsystem1/38(Md62IsTargetPosZone)
  VIPLExitR3LBkReclnUpwdDnwdTrgtPosCalib_TrgtPosArray_read/1 -> [Md27Calib]
  Md27R3LBkReclnUpwdDnwdTrgtPosCalib_TrgtPosArray_read/1 -> [Md14Calib]
  [Md14Calib] -> Subsystem13/3(CalibArray)
  [Pos] -> Subsystem13/2(Pos)
  Subsystem13/2(IsPosZone) -> [Md14IsTargetPosZone]
  Subsystem13/3(IsPosAlready) -> [Md14IsTargetPosAlready]
  [PosDelta] -> Subsystem13/4(Delta)
  [PosTolr] -> Subsystem13/5(Tolr)
  [PosV] -> Subsystem13/1(PosV)
  Subsystem13/1(IsPos) -> [Md14IsTargetPos]
  [Md14IsTargetPos] -> Subsystem1/1(Md14IsTargetPos)
  [Md14IsTargetPosZone] -> Subsystem1/2(Md14IsTargetPosZone)
  [Md14IsTargetPosAlready] -> Subsystem1/3(Md14IsTargetPosAlready)
  [Md14Calib] -> Subsystem/15(Md14Calib)

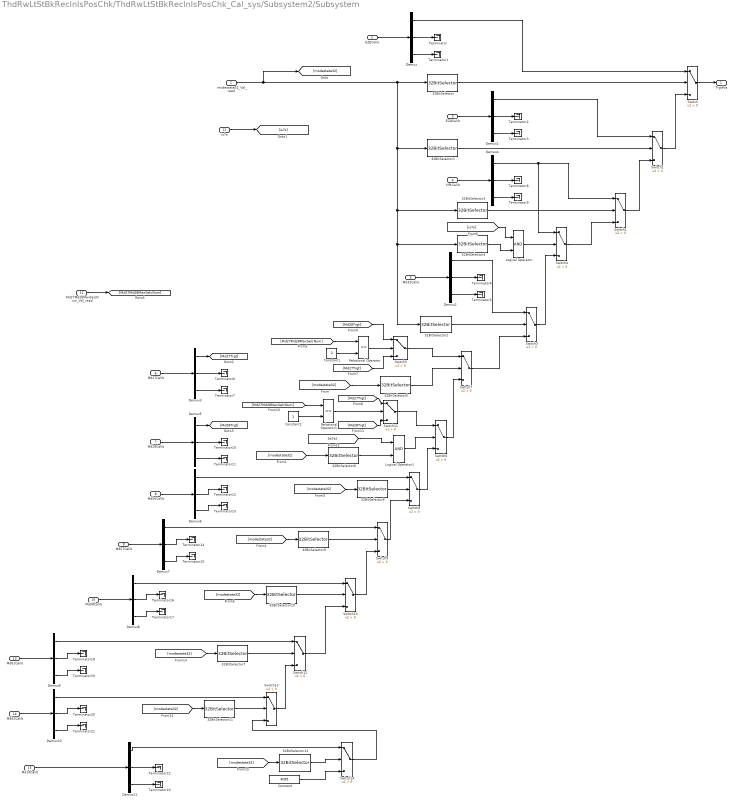
== system ThdRwLtStBkReclnIsPosChk/ThdRwLtStBkReclnIsPosChk_Cal_sys/Subsystem2/Subsystem ==
  modestate32_Val_read : Inport
  EZECalib : Inport  Port=2
  EZQCalib : Inport  Port=3
  VIPLCalib : Inport  Port=4
  Md32Calib : Inport  Port=5
  Md27Calib : Inport  Port=6
  Md28Calib : Inport  Port=7
  Md56Calib : Inport  Port=8
  Md57Calib : Inport  Port=9
  Md58Calib : Inport  Port=10
  is7s : Inport  Port=11
  Md27Md28MaxSelcNum_Val_read : Inport  Port=12
  Md61Calib : Inport  Port=13
  Md62Calib : Inport  Port=14
  Md14Calib : Inport  Port=15
  32BitSelector : StIsPosChkLib/32BitSelector  BitNum=0
  32BitSelector1 : StIsPosChkLib/32BitSelector  BitNum=7
  32BitSelector10 : StIsPosChkLib/32BitSelector  BitNum=21
  32BitSelector11 : StIsPosChkLib/32BitSelector  BitNum=6
  32BitSelector12 : StIsPosChkLib/32BitSelector  BitNum=13
  32BitSelector2 : StIsPosChkLib/32BitSelector  BitNum=31
  32BitSelector3 : StIsPosChkLib/32BitSelector  BitNum=9
  32BitSelector4 : StIsPosChkLib/32BitSelector  BitNum=11
  32BitSelector5 : StIsPosChkLib/32BitSelector  BitNum=26
  32BitSelector6 : StIsPosChkLib/32BitSelector  BitNum=27
  32BitSelector7 : StIsPosChkLib/32BitSelector  BitNum=5
  32BitSelector8 : StIsPosChkLib/32BitSelector  BitNum=24
  32BitSelector9 : StIsPosChkLib/32BitSelector  BitNum=20
  Constant : Constant  Value=4095  OutDataTypeStr=uint16
  Constant1 : Constant  Value=2  OutDataTypeStr=uint8
  Constant2 : Constant  OutDataTypeStr=uint8
  Demux{,1..11} (12 alike) : Demux  Outputs=3
  Logical Operator : Logic  AllPortsSameDT=off  OutDataTypeStr=boolean
  Logical Operator1 : Logic  AllPortsSameDT=off  OutDataTypeStr=boolean
  Relational Operator : RelationalOperator  Operator===  OutDataTypeStr=boolean  RndMeth=Simplest  InputSameDT=off
  Relational Operator1 : RelationalOperator  Operator===  OutDataTypeStr=boolean  RndMeth=Simplest  InputSameDT=off
  Switch{,1..14} (15 alike) : Switch  Criteria=u2 > Threshold  SaturateOnIntegerOverflow=off  InputSameDT=off
  Terminator{,1..23} (24 alike) : Terminator
  TrgtPos : Outport  VectorParamsAs1DForOutWhenUnconnected=off
      settings: EnsureOutportIsVirtual=on
  wires:
  32BitSelector/1 -> Switch/2
  Demux/1 -> Switch/1
  Demux/3 -> Terminator1/1
  Demux/2 -> Terminator/1
  EZECalib/1 -> Demux/1
  EZQCalib/1 -> Demux1/1
  Demux1/2 -> Terminator2/1
  Demux1/3 -> Terminator3/1
  Demux1/1 -> Switch1/1
  Switch/1 -> TrgtPos/1
  Switch1/1 -> Switch/3
  32BitSelector1/1 -> Switch1/2
  Switch4/1 -> Switch2/3
  32BitSelector3/1 -> Switch2/2
  Demux4/3 -> Terminator9/1
  Demux4/2 -> Terminator8/1
  VIPLCalib/1 -> Demux4/1
  Switch2/1 -> Switch1/3
  Demux4/1 -> Switch4/1, Switch2/1
  32BitSelector2/1 -> Switch3/2
  Switch3/1 -> Switch4/3
  modestate32_Val_read/1 -> [modestate32], 32BitSelector2/1, 32BitSelector4/1, 32BitSelector3/1, 32BitSelector1/1, 32BitSelector/1
  Md32Calib/1 -> Demux2/1
  Demux2/2 -> Terminator4/1
  Demux2/3 -> Terminator5/1
  Demux2/1 -> Switch3/1
  Switch7/1 -> Switch3/3
  Switch6/1 -> Switch7/3
  Demux3/3 -> Terminator7/1
  Demux3/2 -> Terminator6/1
  Md27Calib/1 -> Demux3/1
  Md28Calib/1 -> Demux5/1
  Demux5/2 -> Terminator10/1
  Demux5/3 -> Terminator11/1
  [modestate32] -> 32BitSelector5/1
  [modestate32] -> 32BitSelector6/1
  32BitSelector5/1 -> Switch7/2
  Switch8/1 -> Switch6/3
  32BitSelector8/1 -> Switch8/2
  [modestate32] -> 32BitSelector8/1
  Demux6/3 -> Terminator13/1
  Demux6/2 -> Terminator12/1
  Md56Calib/1 -> Demux6/1
  Demux6/1 -> Switch8/1
  Switch9/1 -> Switch8/3
  Switch10/1 -> Switch9/3
  [modestate32] -> 32BitSelector9/1
  32BitSelector9/1 -> Switch9/2
  32BitSelector10/1 -> Switch10/2
  [modestate32] -> 32BitSelector10/1
  Demux7/1 -> Switch9/1
  Md57Calib/1 -> Demux7/1
  Demux7/2 -> Terminator14/1
  Demux7/3 -> Terminator15/1
  Demux8/3 -> Terminator17/1
  Demux8/2 -> Terminator16/1
  Md58Calib/1 -> Demux8/1
  Demux8/1 -> Switch10/1
  is7s/1 -> [is7s]
  Logical Operator/1 -> Switch4/2
  [is7s] -> Logical Operator/1
  32BitSelector4/1 -> Logical Operator/2
  Demux3/1 -> [Md27Trgt]
  Demux5/1 -> [Md28Trgt]
  Md27Md28MaxSelcNum_Val_read/1 -> [Md27Md28MaxSelcNum]
  [Md27Md28MaxSelcNum] -> Relational Operator/1
  Constant1/1 -> Relational Operator/2
  Switch5/1 -> Switch7/1
  Relational Operator/1 -> Switch5/2
  [Md28Trgt] -> Switch5/1
  [Md27Trgt] -> Switch5/3
  Switch11/1 -> Switch6/1
  [Md27Md28MaxSelcNum] -> Relational Operator1/1
  Constant2/1 -> Relational Operator1/2
  Relational Operator1/1 -> Switch11/2
  [Md27Trgt] -> Switch11/1
  [Md28Trgt] -> Switch11/3
  Logical Operator1/1 -> Switch6/2
  32BitSelector6/1 -> Logical Operator1/2
  [is7s] -> Logical Operator1/1
  Demux9/1 -> Switch12/1
  Md61Calib/1 -> Demux9/1
  Demux9/2 -> Terminator18/1
  Demux9/3 -> Terminator19/1
  Demux10/3 -> Terminator21/1
  Demux10/2 -> Terminator20/1
  Md62Calib/1 -> Demux10/1
  Demux10/1 -> Switch13/1
  Switch12/1 -> Switch10/3
  [modestate32] -> 32BitSelector7/1
  32BitSelector7/1 -> Switch12/2
  Switch13/1 -> Switch12/3
  32BitSelector11/1 -> Switch13/2
  [modestate32] -> 32BitSelector11/1
  Demux11/1 -> Switch14/1
  Demux11/2 -> Terminator22/1
  [modestate32] -> 32BitSelector12/1
  Demux11/3 -> Terminator23/1
  Md14Calib/1 -> Demux11/1
  32BitSelector12/1 -> Switch14/2
  Constant/1 -> Switch14/3
  Switch14/1 -> Switch13/3

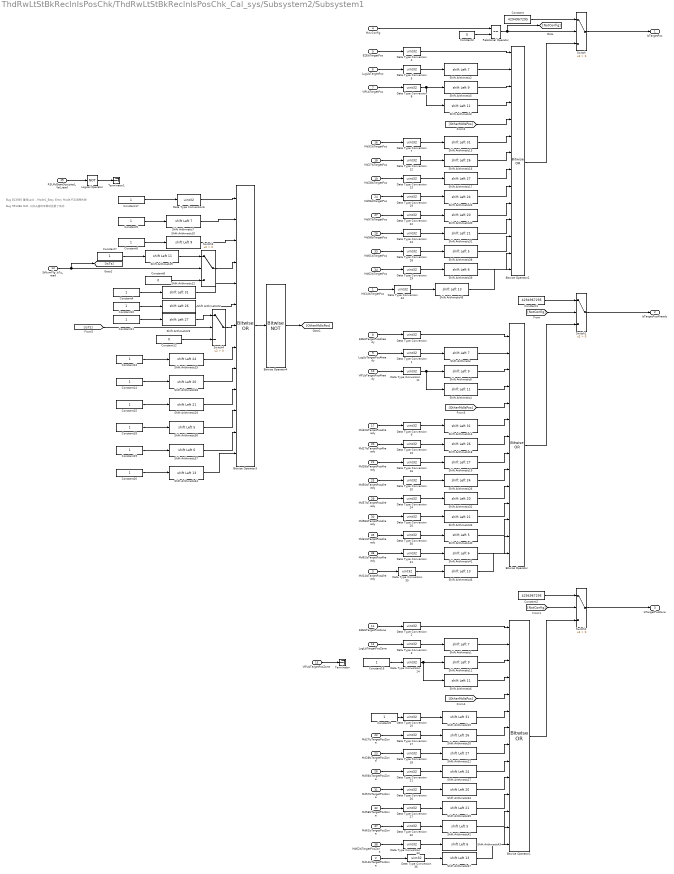
== system ThdRwLtStBkReclnIsPosChk/ThdRwLtStBkReclnIsPosChk_Cal_sys/Subsystem2/Subsystem1 ==
  note: Bug 991386 Md1 三排占座时未移动且报了成功
  note: Bug 813950 童锁Lock，Mode1_Easy Entry Mode 不应调用失败
  Md14IsTargetPos : Inport
  Md14IsTargetPosZone : Inport  Port=2
  Md14IsTargetPosAlready : Inport  Port=3
  MovConfig : Inport  Port=4
  EZEIsTargetPos : Inport  Port=5
  LugLIsTargetPos : Inport  Port=6
  VIPLIsTargetPos : Inport  Port=7
  EZEIsTargetPosAlready : Inport  Port=8
  LugLIsTargetPosAlready : Inport  Port=9
  VIPLIsTargetPosAlready : Inport  Port=10
  EZEIsTargetPosZone : Inport  Port=11
  LugLIsTargetPosZone : Inport  Port=12
  VIPLIsTargetPosZone : Inport  Port=13
  StNumFlg_Is7s_read : Inport  Port=14
  R3LMdSeatOccupied_Val_read : Inport  Port=15
  Md32IsTargetPos : Inport  Port=16
  Md32IsTargetPosAlready : Inport  Port=17
  Md27IsTargetPos : Inport  Port=18
  Md28IsTargetPos : Inport  Port=19
  Md27IsTargetPosAlready : Inport  Port=20
  Md28IsTargetPosAlready : Inport  Port=21
  Md27IsTargetPosZone : Inport  Port=22
  Md28IsTargetPosZone : Inport  Port=23
  Md56IsTargetPos : Inport  Port=24
  Md56IsTargetPosAlready : Inport  Port=25
  Md56IsTargetPosZone : Inport  Port=26
  Md57IsTargetPos : Inport  Port=27
  Md58IsTargetPos : Inport  Port=28
  Md57IsTargetPosAlready : Inport  Port=29
  Md58IsTargetPosAlready : Inport  Port=30
  Md57IsTargetPosZone : Inport  Port=31
  Md58IsTargetPosZone : Inport  Port=32
  Md61IsTargetPos : Inport  Port=33
  Md62IsTargetPos : Inport  Port=34
  Md61IsTargetPosAlready : Inport  Port=35
  Md62IsTargetPosAlready : Inport  Port=36
  Md61IsTargetPosZone : Inport  Port=37
  Md62IsTargetPosZone : Inport  Port=38
  Bitwise Operator : simulink/Logic and Bit Operations/Bitwise Operator  logicop=OR  UseBitMask=off  NumInputPorts=14  BitMask=bin2dec('11011001')  BitMaskRealWorld=Stored Integer
  Bitwise Operator1 : simulink/Logic and Bit Operations/Bitwise Operator  logicop=OR  UseBitMask=off  NumInputPorts=14  BitMask=bin2dec('11011001')  BitMaskRealWorld=Stored Integer
  Bitwise Operator2 : simulink/Logic and Bit Operations/Bitwise Operator  logicop=OR  UseBitMask=off  NumInputPorts=14  BitMask=bin2dec('11011001')  BitMaskRealWorld=Stored Integer
  Bitwise Operator3 : simulink/Logic and Bit Operations/Bitwise Operator  logicop=OR  UseBitMask=off  NumInputPorts=13  BitMask=bin2dec('11011001')  BitMaskRealWorld=Stored Integer
  Bitwise Operator4 : simulink/Logic and Bit Operations/Bitwise Operator  logicop=NOT  UseBitMask=off  BitMask=bin2dec('11011001')  BitMaskRealWorld=Stored Integer
  Constant : Constant  Value=4294967295  OutDataTypeStr=uint32
  Constant1 : Constant  Value=4294967295  OutDataTypeStr=uint32
  Constant{4..7,9..11,13..20} (15 alike) : Constant  OutDataTypeStr=uint32
  Constant12 : Constant  Value=0  OutDataTypeStr=uint32
  Constant2 : Constant  Value=4294967295  OutDataTypeStr=uint32
  Constant3 : Constant  Value=0  OutDataTypeStr=uint8
  Constant8 : Constant  Value=0  OutDataTypeStr=uint32
  Data Type Conversion{,1..36} (37 alike) : DataTypeConversion  OutDataTypeStr=uint32  SaturateOnIntegerOverflow=off  RndMeth=Floor
  Logical Operator : Logic  Operator=NOT  AllPortsSameDT=off  OutDataTypeStr=boolean
  Relational Operator : RelationalOperator  Operator===  OutDataTypeStr=boolean  RndMeth=Simplest  InputSameDT=off
  Shift Arithmetic{,1..2,7} (4 alike) : ArithShift  BitShiftNumber=7  BitShiftDirection=Left
  Shift Arithmetic{5,8,10..11} (4 alike) : ArithShift  BitShiftNumber=9  BitShiftDirection=Left
  Shift Arithmetic{12..15} (4 alike) : ArithShift  BitShiftNumber=31  BitShiftDirection=Left
  Shift Arithmetic{16,18,20,22} (4 alike) : ArithShift  BitShiftNumber=26  BitShiftDirection=Left
  Shift Arithmetic{17,19,21,23} (4 alike) : ArithShift  BitShiftNumber=27  BitShiftDirection=Left
  Shift Arithmetic{24..27} (4 alike) : ArithShift  BitShiftNumber=24  BitShiftDirection=Left
  Shift Arithmetic{28,30,32,34} (4 alike) : ArithShift  BitShiftNumber=20  BitShiftDirection=Left
  Shift Arithmetic{29,31,33,35} (4 alike) : ArithShift  BitShiftNumber=21  BitShiftDirection=Left
  Shift Arithmetic{3..4,6,9} (4 alike) : ArithShift  BitShiftNumber=11  BitShiftDirection=Left
  Shift Arithmetic{36,38,40,42} (4 alike) : ArithShift  BitShiftNumber=5  BitShiftDirection=Left
  Shift Arithmetic{37,39,41,43} (4 alike) : ArithShift  BitShiftNumber=6  BitShiftDirection=Left
  Shift Arithmetic{44..47} (4 alike) : ArithShift  BitShiftNumber=13  BitShiftDirection=Left
  Switch{,1..4} (5 alike) : Switch  Criteria=u2 > Threshold  SaturateOnIntegerOverflow=off  InputSameDT=off
  Terminator : Terminator
  Terminator1 : Terminator
  IsTargetPos : Outport  VectorParamsAs1DForOutWhenUnconnected=off
      settings: EnsureOutportIsVirtual=on
  IsTargetPosAlready : Outport  Port=2  VectorParamsAs1DForOutWhenUnconnected=off
      settings: EnsureOutportIsVirtual=on
  IsTargetPosZone : Outport  Port=3  VectorParamsAs1DForOutWhenUnconnected=off
      settings: EnsureOutportIsVirtual=on
  wires:
  Constant3/1 -> Relational Operator/2
  Constant/1 -> Switch/1
  Relational Operator/1 -> [NotConfig], Switch/2
  MovConfig/1 -> Relational Operator/1
  Switch/1 -> IsTargetPos/1
  [NotConfig] -> Switch1/2
  Constant1/1 -> Switch1/1
  Switch1/1 -> IsTargetPosAlready/1
  Switch2/1 -> IsTargetPosZone/1
  Constant2/1 -> Switch2/1
  [NotConfig] -> Switch2/2
  Data Type Conversion1/1 -> Shift Arithmetic/1
  Data Type Conversion/1 -> Bitwise Operator/1
  Shift Arithmetic/1 -> Bitwise Operator/2
  Shift Arithmetic1/1 -> Bitwise Operator1/2
  Data Type Conversion2/1 -> Bitwise Operator1/1
  Data Type Conversion3/1 -> Shift Arithmetic1/1
  Bitwise Operator1/1 -> Switch2/3
  Bitwise Operator/1 -> Switch1/3
  Shift Arithmetic2/1 -> Bitwise Operator2/2
  Data Type Conversion4/1 -> Bitwise Operator2/1
  Data Type Conversion5/1 -> Shift Arithmetic2/1
  Bitwise Operator2/1 -> Switch/3
  EZEIsTargetPos/1 -> Data Type Conversion4/1
  LugLIsTargetPos/1 -> Data Type Conversion5/1
  LugLIsTargetPosZone/1 -> Data Type Conversion3/1
  EZEIsTargetPosZone/1 -> Data Type Conversion2/1
  LugLIsTargetPosAlready/1 -> Data Type Conversion1/1
  EZEIsTargetPosAlready/1 -> Data Type Conversion/1
  Shift Arithmetic5/1 -> Bitwise Operator2/3
  Data Type Conversion8/1 -> Shift Arithmetic3/1, Shift Arithmetic5/1
  VIPLIsTargetPos/1 -> Data Type Conversion8/1
  VIPLIsTargetPosAlready/1 -> Data Type Conversion11/1
  Data Type Conversion11/1 -> Shift Arithmetic4/1, Shift Arithmetic8/1
  Shift Arithmetic8/1 -> Bitwise Operator/3
  Data Type Conversion14/1 -> Shift Arithmetic6/1, Shift Arithmetic11/1
  Shift Arithmetic11/1 -> Bitwise Operator1/3
  Shift Arithmetic3/1 -> Bitwise Operator2/4
  Shift Arithmetic4/1 -> Bitwise Operator/4
  Shift Arithmetic6/1 -> Bitwise Operator1/4
  Shift Arithmetic10/1 -> Bitwise Operator3/3
  Shift Arithmetic7/1 -> Bitwise Operator3/2
  Constant5/1 -> Shift Arithmetic7/1
  Constant6/1 -> Shift Arithmetic10/1
  Constant7/1 -> Shift Arithmetic9/1
  Bitwise Operator3/1 -> Bitwise Operator4/1
  Bitwise Operator4/1 -> [OtherMdIsPos]
  [OtherMdIsPos] -> Bitwise Operator2/5
  [OtherMdIsPos] -> Bitwise Operator/5
  [OtherMdIsPos] -> Bitwise Operator1/5
  StNumFlg_Is7s_read/1 -> [is7s], Switch3/2
  Shift Arithmetic9/1 -> Switch3/1
  Switch3/1 -> Bitwise Operator3/4
  Constant8/1 -> Switch3/3
  Data Type Conversion6/1 -> Bitwise Operator3/1
  R3LMdSeatOccupied_Val_read/1 -> Logical Operator/1
  Constant4/1 -> Shift Arithmetic12/1
  Shift Arithmetic12/1 -> Bitwise Operator3/5
  Md32IsTargetPos/1 -> Data Type Conversion7/1
  Data Type Conversion7/1 -> Shift Arithmetic13/1
  Shift Arithmetic13/1 -> Bitwise Operator2/6
  Md32IsTargetPosAlready/1 -> Data Type Conversion9/1
  Data Type Conversion9/1 -> Shift Arithmetic14/1
  Shift Arithmetic14/1 -> Bitwise Operator/6
  Constant9/1 -> Data Type Conversion10/1
  Data Type Conversion10/1 -> Shift Arithmetic15/1
  Shift Arithmetic15/1 -> Bitwise Operator1/6
  Md27IsTargetPos/1 -> Data Type Conversion12/1
  Md28IsTargetPos/1 -> Data Type Conversion13/1
  Data Type Conversion12/1 -> Shift Arithmetic16/1
  Data Type Conversion13/1 -> Shift Arithmetic17/1
  Shift Arithmetic16/1 -> Bitwise Operator2/7
  Shift Arithmetic17/1 -> Bitwise Operator2/8
  Md28IsTargetPosAlready/1 -> Data Type Conversion16/1
  Md27IsTargetPosAlready/1 -> Data Type Conversion15/1
  Data Type Conversion15/1 -> Shift Arithmetic18/1
  Data Type Conversion16/1 -> Shift Arithmetic19/1
  Shift Arithmetic18/1 -> Bitwise Operator/7
  Shift Arithmetic19/1 -> Bitwise Operator/8
  Md27IsTargetPosZone/1 -> Data Type Conversion17/1
  Md28IsTargetPosZone/1 -> Data Type Conversion18/1
  Data Type Conversion17/1 -> Shift Arithmetic20/1
  Data Type Conversion18/1 -> Shift Arithmetic21/1
  Shift Arithmetic20/1 -> Bitwise Operator1/7
  Shift Arithmetic21/1 -> Bitwise Operator1/8
  Constant10/1 -> Shift Arithmetic22/1
  Shift Arithmetic22/1 -> Bitwise Operator3/6
  Constant11/1 -> Shift Arithmetic23/1
  Switch4/1 -> Bitwise Operator3/7
  Shift Arithmetic23/1 -> Switch4/1
  [is7s] -> Switch4/2
  Constant12/1 -> Switch4/3
  Shift Arithmetic24/1 -> Bitwise Operator2/9
  Data Type Conversion19/1 -> Shift Arithmetic24/1
  Md56IsTargetPos/1 -> Data Type Conversion19/1
  Shift Arithmetic25/1 -> Bitwise Operator3/8
  Constant13/1 -> Shift Arithmetic25/1
  Shift Arithmetic26/1 -> Bitwise Operator/9
  Data Type Conversion20/1 -> Shift Arithmetic26/1
  Md56IsTargetPosAlready/1 -> Data Type Conversion20/1
  Shift Arithmetic27/1 -> Bitwise Operator1/9
  Data Type Conversion21/1 -> Shift Arithmetic27/1
  Md56IsTargetPosZone/1 -> Data Type Conversion21/1
  Constant14/1 -> Shift Arithmetic28/1
  Shift Arithmetic28/1 -> Bitwise Operator3/9
  Constant15/1 -> Shift Arithmetic29/1
  Shift Arithmetic29/1 -> Bitwise Operator3/10
  Md57IsTargetPos/1 -> Data Type Conversion22/1
  Data Type Conversion22/1 -> Shift Arithmetic30/1
  Shift Arithmetic30/1 -> Bitwise Operator2/10
  Data Type Conversion23/1 -> Shift Arithmetic31/1
  Md58IsTargetPos/1 -> Data Type Conversion23/1
  Shift Arithmetic31/1 -> Bitwise Operator2/11
  Md57IsTargetPosAlready/1 -> Data Type Conversion24/1
  Data Type Conversion24/1 -> Shift Arithmetic32/1
  Shift Arithmetic32/1 -> Bitwise Operator/10
  Shift Arithmetic33/1 -> Bitwise Operator/11
  Data Type Conversion25/1 -> Shift Arithmetic33/1
  Md58IsTargetPosAlready/1 -> Data Type Conversion25/1
  Md57IsTargetPosZone/1 -> Data Type Conversion26/1
  Data Type Conversion26/1 -> Shift Arithmetic34/1
  Shift Arithmetic34/1 -> Bitwise Operator1/10
  Shift Arithmetic35/1 -> Bitwise Operator1/11
  Data Type Conversion27/1 -> Shift Arithmetic35/1
  Md58IsTargetPosZone/1 -> Data Type Conversion27/1
  Constant16/1 -> Data Type Conversion14/1
  VIPLIsTargetPosZone/1 -> Terminator/1
  Constant17/1 -> Data Type Conversion6/1
  Logical Operator/1 -> Terminator1/1
  Constant18/1 -> Shift Arithmetic36/1
  Constant19/1 -> Shift Arithmetic37/1
  Shift Arithmetic36/1 -> Bitwise Operator3/11
  Shift Arithmetic37/1 -> Bitwise Operator3/12
  Shift Arithmetic38/1 -> Bitwise Operator2/12
  Data Type Conversion28/1 -> Shift Arithmetic38/1
  Md61IsTargetPos/1 -> Data Type Conversion28/1
  Md62IsTargetPos/1 -> Data Type Conversion29/1
  Data Type Conversion29/1 -> Shift Arithmetic39/1
  Shift Arithmetic39/1 -> Bitwise Operator2/13
  Md61IsTargetPosAlready/1 -> Data Type Conversion30/1
  Data Type Conversion30/1 -> Shift Arithmetic40/1
  Shift Arithmetic40/1 -> Bitwise Operator/12
  Shift Arithmetic41/1 -> Bitwise Operator/13
  Data Type Conversion31/1 -> Shift Arithmetic41/1
  Md62IsTargetPosAlready/1 -> Data Type Conversion31/1
  Md61IsTargetPosZone/1 -> Data Type Conversion32/1
  Data Type Conversion32/1 -> Shift Arithmetic42/1
  Shift Arithmetic42/1 -> Bitwise Operator1/12
  Shift Arithmetic43/1 -> Bitwise Operator1/13
  Data Type Conversion33/1 -> Shift Arithmetic43/1
  Md62IsTargetPosZone/1 -> Data Type Conversion33/1
  Constant20/1 -> Shift Arithmetic44/1
  Shift Arithmetic44/1 -> Bitwise Operator3/13
  Shift Arithmetic45/1 -> Bitwise Operator2/14
  Data Type Conversion34/1 -> Shift Arithmetic45/1
  Md14IsTargetPos/1 -> Data Type Conversion34/1
  Data Type Conversion35/1 -> Shift Arithmetic46/1
  Md14IsTargetPosAlready/1 -> Data Type Conversion35/1
  Shift Arithmetic46/1 -> Bitwise Operator/14
  Data Type Conversion36/1 -> Shift Arithmetic47/1
  Shift Arithmetic47/1 -> Bitwise Operator1/14
  Md14IsTargetPosZone/1 -> Data Type Conversion36/1

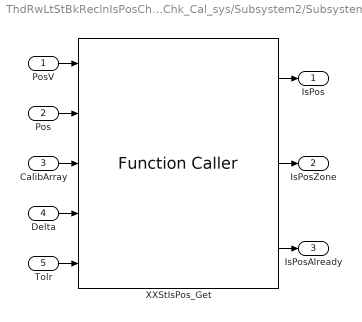
== system ThdRwLtStBkReclnIsPosChk/ThdRwLtStBkReclnIsPosChk_Cal_sys/Subsystem2/Subsystem10 ==
  PosV : Inport
  Pos : Inport  Port=2
  CalibArray : Inport  Port=3
  Delta : Inport  Port=4
  Tolr : Inport  Port=5
  XXStIsPos_Get : FunctionCaller  FunctionPrototype=[IsPos,IsPosZone,IsPosAlready] = XXStIsPos_Get(PosV,Pos,CalibArray,Delta,Tolr)  InputArgumentSpecifications=boolean(true), uint16(1), uint16([1;1;1]), uint16(1), uint16(1)  OutputArgumentSpecifications=boolean(true), boolean(true), boolean(true)
  IsPos : Outport  VectorParamsAs1DForOutWhenUnconnected=off
  IsPosZone : Outport  Port=2  VectorParamsAs1DForOutWhenUnconnected=off
  IsPosAlready : Outport  Port=3  VectorParamsAs1DForOutWhenUnconnected=off
  wires:
  PosV/1 -> XXStIsPos_Get/1
  XXStIsPos_Get/3 -> IsPosAlready/1
  Tolr/1 -> XXStIsPos_Get/5
  XXStIsPos_Get/1 -> IsPos/1
  XXStIsPos_Get/2 -> IsPosZone/1
  CalibArray/1 -> XXStIsPos_Get/3
  Delta/1 -> XXStIsPos_Get/4
  Pos/1 -> XXStIsPos_Get/2

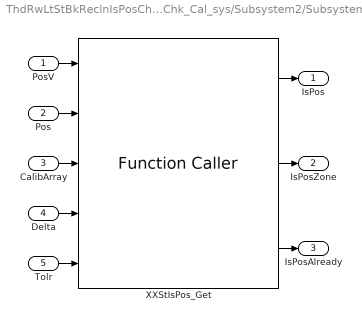
== system ThdRwLtStBkReclnIsPosChk/ThdRwLtStBkReclnIsPosChk_Cal_sys/Subsystem2/Subsystem11 ==
  PosV : Inport
  Pos : Inport  Port=2
  CalibArray : Inport  Port=3
  Delta : Inport  Port=4
  Tolr : Inport  Port=5
  XXStIsPos_Get : FunctionCaller  FunctionPrototype=[IsPos,IsPosZone,IsPosAlready] = XXStIsPos_Get(PosV,Pos,CalibArray,Delta,Tolr)  InputArgumentSpecifications=boolean(true), uint16(1), uint16([1;1;1]), uint16(1), uint16(1)  OutputArgumentSpecifications=boolean(true), boolean(true), boolean(true)
  IsPos : Outport  VectorParamsAs1DForOutWhenUnconnected=off
  IsPosZone : Outport  Port=2  VectorParamsAs1DForOutWhenUnconnected=off
  IsPosAlready : Outport  Port=3  VectorParamsAs1DForOutWhenUnconnected=off
  wires:
  Pos/1 -> XXStIsPos_Get/2
  Delta/1 -> XXStIsPos_Get/4
  CalibArray/1 -> XXStIsPos_Get/3
  XXStIsPos_Get/2 -> IsPosZone/1
  XXStIsPos_Get/1 -> IsPos/1
  Tolr/1 -> XXStIsPos_Get/5
  XXStIsPos_Get/3 -> IsPosAlready/1
  PosV/1 -> XXStIsPos_Get/1

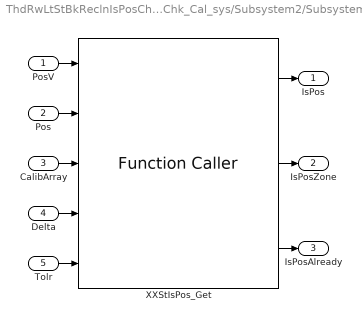
== system ThdRwLtStBkReclnIsPosChk/ThdRwLtStBkReclnIsPosChk_Cal_sys/Subsystem2/Subsystem12 ==
  PosV : Inport
  Pos : Inport  Port=2
  CalibArray : Inport  Port=3
  Delta : Inport  Port=4
  Tolr : Inport  Port=5
  XXStIsPos_Get : FunctionCaller  FunctionPrototype=[IsPos,IsPosZone,IsPosAlready] = XXStIsPos_Get(PosV,Pos,CalibArray,Delta,Tolr)  InputArgumentSpecifications=boolean(true), uint16(1), uint16([1;1;1]), uint16(1), uint16(1)  OutputArgumentSpecifications=boolean(true), boolean(true), boolean(true)
  IsPos : Outport  VectorParamsAs1DForOutWhenUnconnected=off
  IsPosZone : Outport  Port=2  VectorParamsAs1DForOutWhenUnconnected=off
  IsPosAlready : Outport  Port=3  VectorParamsAs1DForOutWhenUnconnected=off
  wires:
  PosV/1 -> XXStIsPos_Get/1
  XXStIsPos_Get/3 -> IsPosAlready/1
  Tolr/1 -> XXStIsPos_Get/5
  XXStIsPos_Get/1 -> IsPos/1
  XXStIsPos_Get/2 -> IsPosZone/1
  CalibArray/1 -> XXStIsPos_Get/3
  Delta/1 -> XXStIsPos_Get/4
  Pos/1 -> XXStIsPos_Get/2

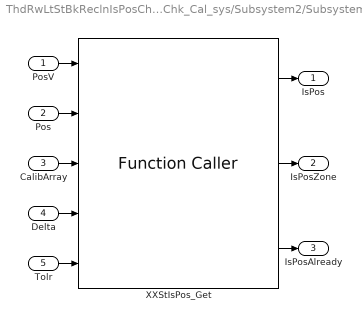
== system ThdRwLtStBkReclnIsPosChk/ThdRwLtStBkReclnIsPosChk_Cal_sys/Subsystem2/Subsystem13 ==
  PosV : Inport
  Pos : Inport  Port=2
  CalibArray : Inport  Port=3
  Delta : Inport  Port=4
  Tolr : Inport  Port=5
  XXStIsPos_Get : FunctionCaller  FunctionPrototype=[IsPos,IsPosZone,IsPosAlready] = XXStIsPos_Get(PosV,Pos,CalibArray,Delta,Tolr)  InputArgumentSpecifications=boolean(true), uint16(1), uint16([1;1;1]), uint16(1), uint16(1)  OutputArgumentSpecifications=boolean(true), boolean(true), boolean(true)
  IsPos : Outport  VectorParamsAs1DForOutWhenUnconnected=off
  IsPosZone : Outport  Port=2  VectorParamsAs1DForOutWhenUnconnected=off
  IsPosAlready : Outport  Port=3  VectorParamsAs1DForOutWhenUnconnected=off
  wires:
  PosV/1 -> XXStIsPos_Get/1
  XXStIsPos_Get/3 -> IsPosAlready/1
  Tolr/1 -> XXStIsPos_Get/5
  XXStIsPos_Get/1 -> IsPos/1
  XXStIsPos_Get/2 -> IsPosZone/1
  CalibArray/1 -> XXStIsPos_Get/3
  Delta/1 -> XXStIsPos_Get/4
  Pos/1 -> XXStIsPos_Get/2
